simulink model "observer"  (R2018a)
settings: Solver=ode23  StartTime=0.0  StopTime=31.8884  RelTol=1e-3
model workspace (MAT data in the model file):
  control : struct (value not decoded)
  input : struct (value not decoded)
  l = 3335
  l1 = 2807
  l2 = 674
  lcontrol = 334
  lt = 665
  output : struct (value not decoded)
  output1 : struct (value not decoded)
  pitch = [-0.00601170594305 0.00114522514384 0.0125445164557 0.0260129427859 0.0413526501937 0.0511756269945 0.0373024628261 0.0532548324432 0.0752374412467 0.0870367972512 0.0703790408797 0.0642023494021 ... (665 elements, 665x1)]
  pitch1 = [0.00235222572609 0.0162413418271 0.0237914073903 0.038703711523 0.0528926975341 0.0693959637901 0.125700648169 0.149036541994 0.168586162345 0.181978559157 0.17648303704 0.173940572128 ... (665 elements, 665x1)]
  roll = [-0.00280308900026 -0.0093555701281 -0.00623960724973 -0.00965013944258 -0.0144960083544 -0.0165739618303 -0.0413451111402 -0.0417587932814 -0.039753610855 -0.0382742391951 -0.0474672160662 -0.0523524236581 ... (665 elements, 665x1)]
  roll1 = [-0.00508976540984 -0.0128769177256 -0.00573808802069 -0.00803683640664 -0.0148569990238 -0.0135250113299 0.00757283220458 0.0108108566268 0.0110824245139 0.0117467287189 0.0115391118445 0.00812049366445 ... (665 elements, 665x1)]
  rtk_P = [0 0 0.00725817699424 0.00725817699424 -4.192609801e-16 -4.192609801e-16 0.00725817698288 0.00725817698288 -6.06069014419e-17 -6.06069014419e-17 0.00725817697152 0.00725817697152 ... (2022 elements, 674x3)]
  simin : struct (value not decoded)
  t = [85.2681087899 153.847078989 135.937655107 145.710208503 139.738803374 143.646452387 141.245887466 142.795164057 141.986419874 142.477492231 142.340892456 142.389396391 ... (674 elements, 674x1)]
  temp = [0.000186264650653 -0.000333016556148 0.00127742410264 0.00224038281138 0.00429726594319 -0.00123745127094 -0.0498635877438 -0.0654781132175 -0.0797628012916 -0.0994190421594 -0.130389530625 -0.157448428987 ... (674 elements, 674x1)]
  time = [137013148 137105522 137113114 137205498 137213142 137305502 137313143 137385536 137393177 137505497 137513125 137605502 ... (665 elements, 665x1)]
  tout = [0 40 80 120 160 200 240 280 320 360 400 440 ... (51 elements, 51x1)]
  ups = [-0.00390798864963 -0.0343320965106 -0.0636578539957 -0.075087173802 -0.0805963166531 -0.0991310672402 -0.125807682301 -0.141612416937 -0.141039897482 -0.132345709554 -0.120718475957 -0.105525554245 ... (665 elements, 665x1)]
  urs = [-0.0193064957453 -0.00988556947443 0.00896900324588 0.0192245887848 0.0131872654637 -0.000864770461033 -0.0106332547779 -0.00981483295256 -0.00119475892361 0.00693320512295 0.00799889781381 0.00317561720843 ... (665 elements, 665x1)]
  uts = [0.664106860951 0.749481484877 0.672099541838 0.648171853238 0.700691335264 0.708512249166 0.659850468498 0.640879189244 0.664961763399 0.668205140062 0.640989688844 0.625700347079 ... (665 elements, 665x1)]
  uys = [0.0139395447601 0.0198481563309 0.0256425224772 0.0339606547853 0.0446716994275 0.0544470884218 0.06301463774 0.0718767917399 0.0826736407 0.0943232231429 0.10641126735 0.11853603151 ... (665 elements, 665x1)]
  x = [8.71560944851e-05 -0.000263895544732 0.000265805954332 0.000300014003894 0.000591371497193 0.000529778841884 0.00684193504836 0.00668914061072 0.00254694811157 -0.00143805981445 -0.0136823182856 -0.0178010839904 ... (665 elements, 665x1)]
  x1 = [8.54283814042e-05 -0.000351541918258 0.000561343727981 0.00122062991294 0.00226118745505 0.0017878063312 -0.0048216263535 -0.0106732543262 -0.0180693220189 -0.0278330591582 -0.0298109986026 -0.0413157469741 ... (665 elements, 665x1)]
  x_av = [8.62922379446e-05 -0.000307718731495 0.000413574841157 0.000760321958416 0.00142627947612 0.00115879258654 0.00101015434743 -0.00199205685772 -0.00776118695365 -0.0146355594863 -0.0217466584441 -0.0295584154823 ... (665 elements, 665x1)]
  xt = [-6.06069014419e-17 0.00725817697152 0.00725817697152 -5.47955244547e-11 -5.47955244547e-11 -5.57118682784e-11 -5.57118682784e-11 -0.00725817702815 -0.00725817702815 -0.0145163542274 -0.0145163542274 -0.0290327088019 ... (665 elements, 665x1)]
  y = [4.71199364932e-05 -0.000202451032641 0.00110205359743 0.00274075291804 0.00386317545071 0.0039759501557 0.0111320604636 0.0200674919449 0.0256167559869 0.0328388617799 0.00902856975366 0.0187732326011 ... (665 elements, 665x1)]
  y1 = [0.000186264650653 -0.000333016556148 0.00127742410264 0.00224038281138 0.00429726594319 -0.00123745127094 -0.0498635877438 -0.0654781132175 -0.0797628012916 -0.0994190421594 -0.130389530625 -0.157448428987 ... (665 elements, 665x1)]
  y_av = [0.000116692293573 -0.000267733794395 0.00118973885004 0.00249056786471 0.00408022069695 0.00136924944238 -0.0193657636401 -0.0227053106363 -0.0270730226523 -0.0332900901898 -0.0606804804357 -0.0693375981928 ... (665 elements, 665x1)]
  yaw = [0.551630744054 0.985953522054 0.860467849076 0.912170384354 0.864267212524 0.877979115519 0.85252446167 0.850917442274 0.835099319744 0.825993656962 0.8192363021 0.809230396231 ... (665 elements, 665x1)]
  yaw1 = [0.524311158471 0.914078236382 0.795656408279 0.841193934159 0.796803282272 0.809519389357 0.787366234758 0.785910630038 0.771945888619 0.763168855651 0.757543515422 0.745155737898 ... (665 elements, 665x1)]
  yt = [2.07646400074e-15 -8.22783768201e-10 -8.22783768201e-10 -0.0111218847698 -0.0111218847698 -0.0222437696223 -0.0222437696223 -0.0333656546197 -0.0333656546197 -0.0444875400883 -0.0444875400883 -0.0667313107556 ... (665 elements, 665x1)]
  z = [-0.0994666679592 -0.214162644666 -0.215226967159 -0.256145303395 -0.292239651406 -0.309925352113 -0.350361829325 -0.36096245045 -0.394865238248 -0.398678408621 -0.417742992449 -0.417553654594 ... (674 elements, 674x1)]
  z1 = [-0.103229820714 -0.203136396463 -0.194407590044 -0.247819005734 -0.277075354685 -0.291884441153 -0.321788426104 -0.334001860067 -0.367445284083 -0.368818531247 -0.415153871284 -0.416306471083 ... (674 elements, 674x1)]
(part 2 of 2)

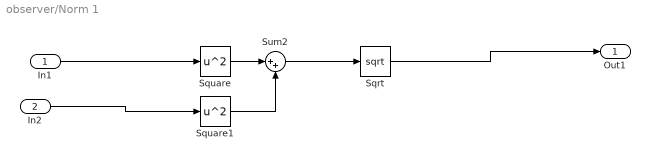
== system observer/Norm 1 ==
  In1 : Inport
  In2 : Inport  Port=2
  Sqrt : Sqrt  SaturateOnIntegerOverflow=on
  Square : Math  Operator=square  SaturateOnIntegerOverflow=on
  Square1 : Math  Operator=square  SaturateOnIntegerOverflow=on
  Sum2 : Sum  Inputs=|++
  Out1 : Outport
  wires:
  Sum2/1 -> Sqrt/1
  Square1/1 -> Sum2/2
  Square/1 -> Sum2/1
  In2/1 -> Square1/1
  Sqrt/1 -> Out1/1
  In1/1 -> Square/1

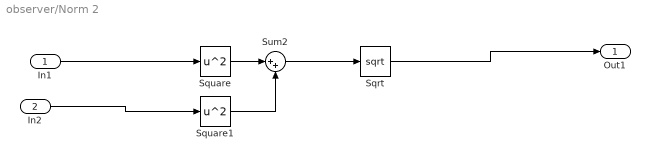
== system observer/Norm 2 ==
  In1 : Inport
  In2 : Inport  Port=2
  Sqrt : Sqrt  SaturateOnIntegerOverflow=on
  Square : Math  Operator=square  SaturateOnIntegerOverflow=on
  Square1 : Math  Operator=square  SaturateOnIntegerOverflow=on
  Sum2 : Sum  Inputs=|++
  Out1 : Outport
  wires:
  Sum2/1 -> Sqrt/1
  Square1/1 -> Sum2/2
  Square/1 -> Sum2/1
  In2/1 -> Square1/1
  Sqrt/1 -> Out1/1
  In1/1 -> Square/1

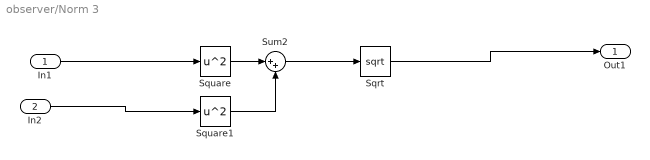
== system observer/Norm 3 ==
  In1 : Inport
  In2 : Inport  Port=2
  Sqrt : Sqrt  SaturateOnIntegerOverflow=on
  Square : Math  Operator=square  SaturateOnIntegerOverflow=on
  Square1 : Math  Operator=square  SaturateOnIntegerOverflow=on
  Sum2 : Sum  Inputs=|++
  Out1 : Outport
  wires:
  Sum2/1 -> Sqrt/1
  Square1/1 -> Sum2/2
  Square/1 -> Sum2/1
  In2/1 -> Square1/1
  Sqrt/1 -> Out1/1
  In1/1 -> Square/1

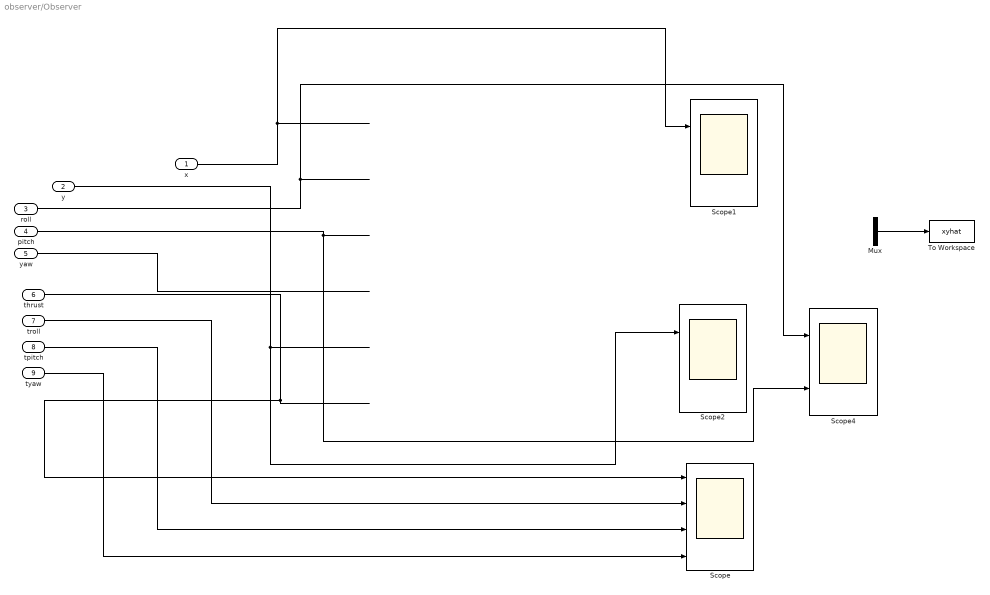
== system observer/Observer  ==
  x : Inport
  y : Inport  Port=2
  roll : Inport  Port=3
  pitch : Inport  Port=4
  yaw : Inport  Port=5
  thrust : Inport  Port=6
  troll : Inport  Port=7
  tpitch : Inport  Port=8
  tyaw : Inport  Port=9
  Mux : Mux  Inputs=2
  Scope : Scope  NumInputPorts=4
  Scope1 : Scope  NumInputPorts=2
  Scope2 : Scope  NumInputPorts=2
  Scope4 : Scope  NumInputPorts=2
  To Workspace : ToWorkspace  VariableName=xyhat  SampleTime=0.01
  wires:
  y/1 -> Scope2/1
  pitch/1 -> Scope4/2
  tyaw/1 -> Scope/4
  ? -> Scope1/2, Mux/1
  ? -> Mux/2, Scope2/2  "yhat"
  thrust/1 -> Scope/1
  roll/1 -> Scope4/1
  troll/1 -> Scope/2
  Mux/1 -> To Workspace/1
  x/1 -> Scope1/1
  yaw/1 -> ?
  tpitch/1 -> Scope/3
